simulink model "PMLSM_ThreeLoop_Simple"  (R2026b)
settings: Solver=FixedStepDiscrete  StopTime=12  FixedStep=PMLSM_Ts_s
PreLoadFcn:
  | init_PMLSM_fpga_cosim_params;
InitFcn:
  | reload(get_param('PMLSM_ThreeLoop_Simple','ModelWorkspace'));
values from neighbouring files (symbols this model uses):
  CPU_Clock = 200e6    (= 200000000)    [PMSLM_Init_Params_MBDL4.m]
  FPGA_Cosim_Enable = 1    [init_PMLSM_fpga_cosim_params.m]
  FPGA_Cosim_Input_Mode = 1    [init_PMLSM_fpga_cosim_params.m]
  FPGA_Cosim_Ts_s = 50e-6    (= 5e-05)    [init_PMLSM_fpga_cosim_params.m]
  FPGA_Reference_Mode = 1    [init_PMLSM_step7c_params.m]
  FPGA_Smoke_ia_A = 1.0    (= 1)    [init_PMLSM_fpga_cosim_params.m]
  FPGA_Smoke_ib_A = -0.5    [init_PMLSM_fpga_cosim_params.m]
  FPGA_Smoke_ic_A = -0.5    [init_PMLSM_fpga_cosim_params.m]
  FPGA_Smoke_id_ref_A = 0.0    (= 0)    [init_PMLSM_fpga_cosim_params.m]
  FPGA_Smoke_iq_ref_A = 0.0    (= 0)    [init_PMLSM_fpga_cosim_params.m]
  FPGA_Smoke_theta_rad = 0.0    (= 0)    [init_PMLSM_fpga_cosim_params.m]
  FPGA_Smoke_vdc_V = 48.0    (= 48)    [init_PMLSM_fpga_cosim_params.m]
  FPGA_Smoke_we_radps = 0.0    (= 0)    [init_PMLSM_fpga_cosim_params.m]
  FPGA_TBPRD = 2500    [init_PMLSM_fpga_cosim_params.m]
  Iq_fric_run = 0.05    [PMSLM_Init_Params_MBDL4.m]
  Iq_fric_start = 0.40    (= 0.4)    [PMSLM_Init_Params_MBDL4.m]
  Iq_int_limit = 0.10    (= 0.1)    [PMSLM_Init_Params_MBDL4.m]
  Kaw_d = Kaw_q    (= 0.2)    [PMSLM_Init_Params_MBDL4.m]
  Kaw_q = 0.2    [PMSLM_Init_Params_MBDL4.m]
  Kaw_s = 0.4    [PMSLM_Init_Params_MBDL4.m]
  Ki_ACR = ACR_Commissioning_Scale*Ki_ACR_Baseline    (= 2962.5)    [PMSLM_Init_Params_MBDL4.m]
  Ki_ASR = 0.05    [PMSLM_Init_Params_MBDL4.m]
  Kp_ACR = ACR_Commissioning_Scale*Kp_ACR_Baseline    (= 2.18125)    [PMSLM_Init_Params_MBDL4.m]
  Kp_ASR = 0.03    [PMSLM_Init_Params_MBDL4.m]
  Kp_pos = 5    [PMSLM_Init_Params_MBDL4.m]
  PMLSM_Ld_H = Ld    (= 0.001745)    [PMSLM_Init_Params_MBDL4.m]
  PMLSM_Lq_H = Lq    (= 0.001745)    [PMSLM_Init_Params_MBDL4.m]
  PMLSM_psi_f_Wb = flux    (= 0.141)    [PMSLM_Init_Params_MBDL4.m]
  PMLSM_Rs_ohm = Rs    (= 2.37)    [PMSLM_Init_Params_MBDL4.m]
  Pos_deadband = 0.02    [PMSLM_Init_Params_MBDL4.m]
  Speed_loop_Iq_Limit = Iq_Limit    (= 0.3)    [PMSLM_Init_Params_MBDL4.m]
  Ts = 1 / PWM_Freq    (= 0.0001)    [PMSLM_Init_Params_MBDL4.m]
  Ts_ACR = 1e-4    (= 0.0001)    [PMSLM_Init_Params_MBDL4.m]
  Ts_ASR = 1e-3    (= 0.001)    [PMSLM_Init_Params_MBDL4.m]
  Udc = 48    [PMSLM_Init_Params_MBDL4.m]
  v_ff_eps = 0.5    [PMSLM_Init_Params_MBDL4.m]
  v_over_eps = 3    [PMSLM_Init_Params_MBDL4.m]
  V_pos_max_mmps = 10    [PMSLM_Init_Params_MBDL4.m]
  v_ref_max = 20    [PMSLM_Init_Params_MBDL4.m]
  v_ref_set_step_dn = v_ref_set_rate_dn * Ts    (= 0.005)    [PMSLM_Init_Params_MBDL4.m]
  v_ref_set_step_up = v_ref_set_rate_up * Ts    (= 0.005)    [PMSLM_Init_Params_MBDL4.m]
  v_ref_zero_eps = 0.2    [PMSLM_Init_Params_MBDL4.m]
  v_stick_off = 3.0    (= 3)    [PMSLM_Init_Params_MBDL4.m]
  v_stick_on = 1.0    (= 1)    [PMSLM_Init_Params_MBDL4.m]
undefined symbols (not defined in the file or in its folder): DiscIntNeverNeededParam, Host_Enable_Schedule, Host_Id_A, Host_Iq_A, Host_Iq_Test_Mode, Host_Load_N, Host_PI_Reset_EN, Host_Speed_mmps, Host_Speed_Ramp_s, Host_Start_s, Host_Target_mm, Host_Traj_Amax, Host_Traj_Jmax, Host_Traj_Vmax, PMLSM_Bv_N_per_mps, PMLSM_deadtime_current_eps_A, PMLSM_deadtime_ratio, PMLSM_Fc_N, PMLSM_Kf_peak_N_per_Apeak, PMLSM_M_kg, PMLSM_pwm_period_counts, PMLSM_tau_NN_m, PMLSM_theta_offset_rad, PMLSM_Ts_s, PMLSM_v_eps_mps
libraries: simulink x7, mcbeeMathTransformLib x2, vivadosimlib x1
(part 1 of 2)

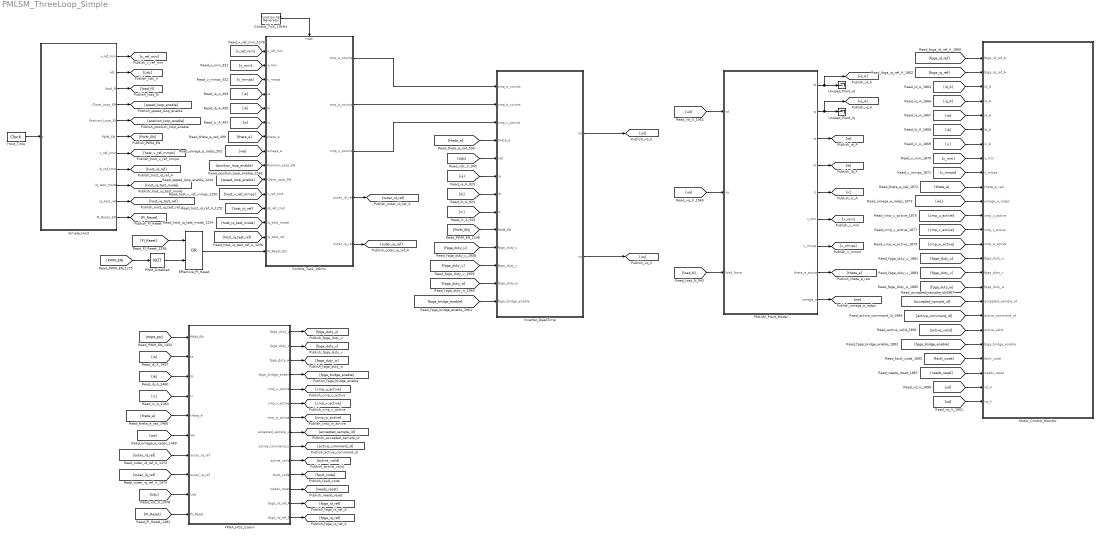
== system PMLSM_ThreeLoop_Simple ==
  Control_Task_10kHz : Subsystem
  Control_Tick_10kHz : FunctionCallGenerator  SampleTime=Ts
  Effective_PI_Reset : Logic  Operator=OR  AllPortsSameDT=off  OutDataTypeStr=boolean
  FPGA_HDL_Cosim : Subsystem
  Host_Time : DigitalClock  SampleTime=Ts_ACR
  Inverter_DeadTime : Subsystem
  Motor_Control_Monitor : Subsystem
  PMLSM_Plant_Model : Subsystem
  PWM_Disabled : Logic  Operator=NOT  AllPortsSameDT=off  OutDataTypeStr=boolean
  Simple_Host : MATLAB Function  TreatAsAtomicUnit=on
  Unused_Plant_Id : Terminator
  Unused_Plant_Iq : Terminator
  wires:
  Host_Time/1 -> Simple_Host/1(t)
  Simple_Host/2(vdc) -> [Udc]
  Simple_Host/3(load_N) -> [load_N]
  Simple_Host/11(PI_Reset_EN) -> [PI_Reset]
  Simple_Host/10(iq_test_ref) -> [host_iq_test_ref]
  Simple_Host/9(iq_test_mode) -> [host_iq_test_mode]
  Simple_Host/8(id_ref_cmd) -> [host_id_ref]
  Simple_Host/7(v_ref_cmd) -> [host_v_ref_mmps]
  Simple_Host/6(PWM_EN) -> [PWM_EN]
  Simple_Host/5(Position_Loop_EN) -> [position_loop_enable]
  Simple_Host/4(Close_Loop_EN) -> [speed_loop_enable]
  [PWM_EN] -> PWM_Disabled/1
  PWM_Disabled/1 -> Effective_PI_Reset/2
  Effective_PI_Reset/1 -> Control_Task_10kHz/15(PI_Reset_EN)
  [speed_loop_enable] -> Control_Task_10kHz/10(Close_Loop_EN)
  [position_loop_enable] -> Control_Task_10kHz/9(Position_Loop_EN)
  [host_v_ref_mmps] -> Control_Task_10kHz/11(v_ref_cmd)
  [host_id_ref] -> Control_Task_10kHz/12(id_ref_cmd)
  [host_iq_test_mode] -> Control_Task_10kHz/13(iq_test_mode)
  [host_iq_test_ref] -> Control_Task_10kHz/14(iq_test_ref)
  [PI_Reset] -> Effective_PI_Reset/1
  Simple_Host/1(x_ref_mm) -> [x_ref_mm]
  [x_mm] -> Control_Task_10kHz/2(x_mm)
  [v_mmps] -> Control_Task_10kHz/3(v_mmps)
  [ia] -> Control_Task_10kHz/4(ia)
  [ib] -> Control_Task_10kHz/5(ib)
  [ic] -> Control_Task_10kHz/6(ic)
  [we] -> Control_Task_10kHz/8(omega_e)
  [theta_e] -> Control_Task_10kHz/7(theta_e)
  Control_Tick_10kHz/1 -> Control_Task_10kHz/Trigger
  [x_ref_mm] -> Control_Task_10kHz/1(x_ref_mm)
  [uq] -> Motor_Control_Monitor/25(vq_V)
  [ud] -> Motor_Control_Monitor/24(vd_V)
  [needs_reset] -> Motor_Control_Monitor/23(needs_reset)
  [fault_code] -> Motor_Control_Monitor/22(fault_code)
  [fpga_bridge_enable] -> Motor_Control_Monitor/21(fpga_bridge_enable)
  [active_valid] -> Motor_Control_Monitor/20(active_valid)
  [active_command_id] -> Motor_Control_Monitor/19(active_command_id)
  [accepted_sample_id] -> Motor_Control_Monitor/18(accepted_sample_id)
  [fpga_duty_w] -> Motor_Control_Monitor/17(fpga_duty_w)
  [fpga_duty_v] -> Motor_Control_Monitor/16(fpga_duty_v)
  [fpga_duty_u] -> Motor_Control_Monitor/15(fpga_duty_u)
  [cmp_w_active] -> Motor_Control_Monitor/14(cmp_w_active)
  [cmp_v_active] -> Motor_Control_Monitor/13(cmp_v_active)
  [cmp_u_active] -> Motor_Control_Monitor/12(cmp_u_active)
  [we] -> Motor_Control_Monitor/11(omega_e_radps)
  [theta_e] -> Motor_Control_Monitor/10(theta_e_rad)
  [v_mmps] -> Motor_Control_Monitor/9(v_mmps)
  [x_mm] -> Motor_Control_Monitor/8(x_mm)
  [ic] -> Motor_Control_Monitor/7(ic_A)
  [ib] -> Motor_Control_Monitor/6(ib_A)
  [ia] -> Motor_Control_Monitor/5(ia_A)
  [iq_A] -> Motor_Control_Monitor/4(iq_A)
  [id_A] -> Motor_Control_Monitor/3(id_A)
  [fpga_iq_ref] -> Motor_Control_Monitor/2(fpga_iq_ref_A)
  [fpga_id_ref] -> Motor_Control_Monitor/1(fpga_id_ref_A)
  FPGA_HDL_Cosim/12(needs_reset) -> [needs_reset]
  FPGA_HDL_Cosim/11(fault_code) -> [fault_code]
  FPGA_HDL_Cosim/10(active_valid) -> [active_valid]
  FPGA_HDL_Cosim/9(active_command_id) -> [active_command_id]
  FPGA_HDL_Cosim/8(accepted_sample_id) -> [accepted_sample_id]
  FPGA_HDL_Cosim/7(cmp_w_active) -> [cmp_w_active]
  FPGA_HDL_Cosim/6(cmp_v_active) -> [cmp_v_active]
  FPGA_HDL_Cosim/5(cmp_u_active) -> [cmp_u_active]
  FPGA_HDL_Cosim/14(fpga_iq_ref_A) -> [fpga_iq_ref]
  FPGA_HDL_Cosim/13(fpga_id_ref_A) -> [fpga_id_ref]
  FPGA_HDL_Cosim/4(fpga_bridge_enable) -> [fpga_bridge_enable]
  FPGA_HDL_Cosim/3(fpga_duty_w) -> [fpga_duty_w]
  FPGA_HDL_Cosim/2(fpga_duty_v) -> [fpga_duty_v]
  FPGA_HDL_Cosim/1(fpga_duty_u) -> [fpga_duty_u]
  [PI_Reset] -> FPGA_HDL_Cosim/10(PI_Reset)
  [Udc] -> FPGA_HDL_Cosim/9(Udc)
  [outer_iq_ref] -> FPGA_HDL_Cosim/8(outer_iq_ref)
  [outer_id_ref] -> FPGA_HDL_Cosim/7(outer_id_ref)
  [we] -> FPGA_HDL_Cosim/6(we)
  [theta_e] -> FPGA_HDL_Cosim/5(theta_e)
  [ic] -> FPGA_HDL_Cosim/4(ic)
  [ib] -> FPGA_HDL_Cosim/3(ib)
  [ia] -> FPGA_HDL_Cosim/2(ia)
  [PWM_EN] -> FPGA_HDL_Cosim/1(PWM_EN)
  PMLSM_Plant_Model/6(x_mm) -> [x_mm]
  PMLSM_Plant_Model/7(v_mmps) -> [v_mmps]
  PMLSM_Plant_Model/3(ia) -> [ia]
  PMLSM_Plant_Model/4(ib) -> [ib]
  PMLSM_Plant_Model/5(ic) -> [ic]
  PMLSM_Plant_Model/8(theta_e_actual) -> [theta_e]
  PMLSM_Plant_Model/9(omega_e) -> [we]
  PMLSM_Plant_Model/1(id) -> Unused_Plant_Id/1, [id_A]
  PMLSM_Plant_Model/2(iq) -> Unused_Plant_Iq/1, [iq_A]
  [load_N] -> PMLSM_Plant_Model/3(load_force)
  Control_Task_10kHz/5(outer_iq_ref) -> [outer_iq_ref]
  Control_Task_10kHz/4(outer_id_ref) -> [outer_id_ref]
  [uq] -> PMLSM_Plant_Model/2(vq)
  [ud] -> PMLSM_Plant_Model/1(vd)
  [fpga_bridge_enable] -> Inverter_DeadTime/13(fpga_bridge_enable)
  [fpga_duty_w] -> Inverter_DeadTime/12(fpga_duty_w)
  [fpga_duty_v] -> Inverter_DeadTime/11(fpga_duty_v)
  [fpga_duty_u] -> Inverter_DeadTime/10(fpga_duty_u)
  [ic] -> Inverter_DeadTime/8(ic)
  [ib] -> Inverter_DeadTime/7(ib)
  [ia] -> Inverter_DeadTime/6(ia)
  [theta_e] -> Inverter_DeadTime/4(theta_e)
  [Udc] -> Inverter_DeadTime/5(vdc)
  Inverter_DeadTime/1(vd) -> [ud]
  Inverter_DeadTime/2(vq) -> [uq]
  [PWM_EN] -> Inverter_DeadTime/9(PWM_EN)
  Control_Task_10kHz/1(cmp_a_counts) -> Inverter_DeadTime/1(cmp_a_counts)
  Control_Task_10kHz/2(cmp_b_counts) -> Inverter_DeadTime/2(cmp_b_counts)
  Control_Task_10kHz/3(cmp_c_counts) -> Inverter_DeadTime/3(cmp_c_counts)

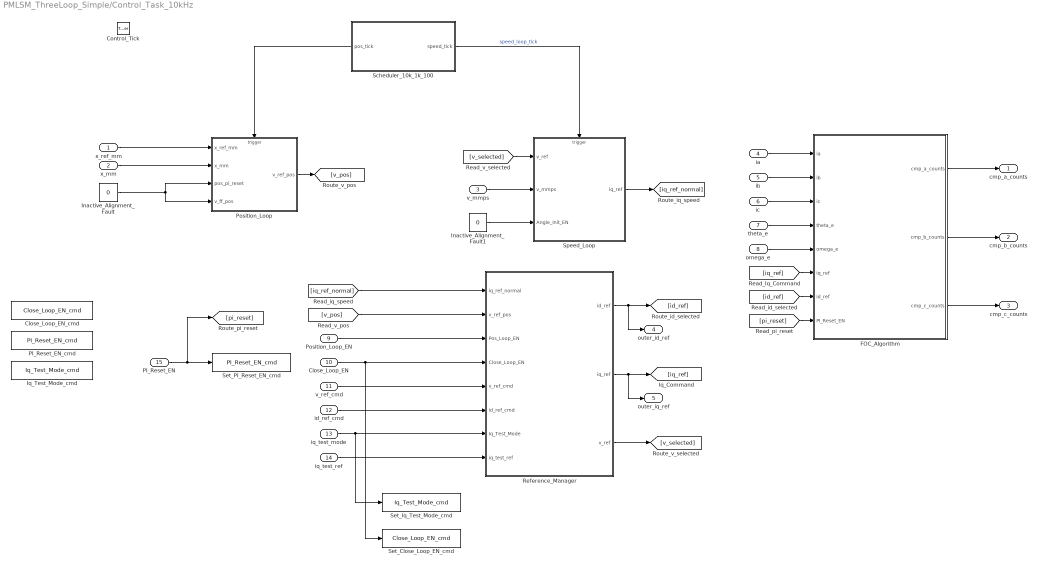
== system PMLSM_ThreeLoop_Simple/Control_Task_10kHz ==
  x_ref_mm : Inport
  x_mm : Inport  Port=2
  v_mmps : Inport  Port=3
  ia : Inport  Port=4
  ib : Inport  Port=5
  ic : Inport  Port=6
  theta_e : Inport  Port=7
  omega_e : Inport  Port=8
  Position_Loop_EN : Inport  Port=9
  Close_Loop_EN : Inport  Port=10
  v_ref_cmd : Inport  Port=11
  id_ref_cmd : Inport  Port=12
  iq_test_mode : Inport  Port=13
  iq_test_ref : Inport  Port=14
  PI_Reset_EN : Inport  Port=15
  Control_Tick : TriggerPort  TriggerType=function-call  VariantControl=(inherit)  PortDimensions=1
  Close_Loop_EN_cmd : DataStoreMemory  DataStoreName=Close_Loop_EN_cmd  WriteAfterWriteMsg=warning  InitialValue=1  ShowAdditionalParam=off
  FOC_Algorithm : Subsystem
  Inactive_Alignment_Fault : Constant  Value=0
  Inactive_Alignment_Fault1 : Constant  Value=0
  Iq_Test_Mode_cmd : DataStoreMemory  DataStoreName=Iq_Test_Mode_cmd  WriteAfterWriteMsg=warning  ShowAdditionalParam=off
  PI_Reset_EN_cmd : DataStoreMemory  DataStoreName=PI_Reset_EN_cmd  WriteAfterWriteMsg=warning  ShowAdditionalParam=off
  Position_Loop : Subsystem  TreatAsAtomicUnit=on
  Reference_Manager : Subsystem
  Scheduler_10k_1k_100 : Subsystem
  Set_Close_Loop_EN_cmd : DataStoreWrite  Priority=-10  DataStoreName=Close_Loop_EN_cmd  IndexOptions=Index vector (dialog)  Indices=1  OutputSizes=1
  Set_Iq_Test_Mode_cmd : DataStoreWrite  Priority=-10  DataStoreName=Iq_Test_Mode_cmd  IndexOptions=Index vector (dialog)  Indices=1  OutputSizes=1
  Set_PI_Reset_EN_cmd : DataStoreWrite  Priority=-10  DataStoreName=PI_Reset_EN_cmd  IndexOptions=Index vector (dialog)  Indices=1  OutputSizes=1
  Speed_Loop : Subsystem  TreatAsAtomicUnit=on
  cmp_a_counts : Outport
  cmp_b_counts : Outport  Port=2
  cmp_c_counts : Outport  Port=3
  outer_id_ref : Outport  Port=4
  outer_iq_ref : Outport  Port=5
  wires:
  [iq_ref] -> FOC_Algorithm/6(iq_ref)
  FOC_Algorithm/3(cmp_c_counts) -> cmp_c_counts/1
  FOC_Algorithm/2(cmp_b_counts) -> cmp_b_counts/1
  FOC_Algorithm/1(cmp_a_counts) -> cmp_a_counts/1
  omega_e/1 -> FOC_Algorithm/5(omega_e)
  theta_e/1 -> FOC_Algorithm/4(theta_e)
  ic/1 -> FOC_Algorithm/3(ic)
  ib/1 -> FOC_Algorithm/2(ib)
  ia/1 -> FOC_Algorithm/1(ia)
  iq_test_ref/1 -> Reference_Manager/8(iq_test_ref)
  id_ref_cmd/1 -> Reference_Manager/6(id_ref_cmd)
  v_ref_cmd/1 -> Reference_Manager/5(v_ref_cmd)
  Position_Loop_EN/1 -> Reference_Manager/3(Pos_Loop_EN)
  [pi_reset] -> FOC_Algorithm/8(PI_Reset_EN)
  [id_ref] -> FOC_Algorithm/7(id_ref)
  [v_selected] -> Speed_Loop/1(v_ref)
  [iq_ref_normal] -> Reference_Manager/1(iq_ref_normal)
  [v_pos] -> Reference_Manager/2(v_ref_pos)
  Reference_Manager/3(v_ref) -> [v_selected]
  Inactive_Alignment_Fault/1 -> Position_Loop/3(pos_pi_reset), Position_Loop/4(v_ff_pos)
  Speed_Loop/1(iq_ref) -> [iq_ref_normal]
  Position_Loop/1(v_ref_pos) -> [v_pos]
  x_mm/1 -> Position_Loop/2(x_mm)
  x_ref_mm/1 -> Position_Loop/1(x_ref_mm)
  Scheduler_10k_1k_100/1(speed_tick) -> Speed_Loop/Trigger  "speed_loop_tick"
  Scheduler_10k_1k_100/2(pos_tick) -> Position_Loop/Trigger
  PI_Reset_EN/1 -> [pi_reset], Set_PI_Reset_EN_cmd/1
  iq_test_mode/1 -> Set_Iq_Test_Mode_cmd/1, Reference_Manager/7(Iq_Test_Mode)
  Close_Loop_EN/1 -> Set_Close_Loop_EN_cmd/1, Reference_Manager/4(Close_Loop_EN)
  Inactive_Alignment_Fault1/1 -> Speed_Loop/3(Angle_Init_EN)
  v_mmps/1 -> Speed_Loop/2(v_mmps)
  Reference_Manager/1(id_ref) -> outer_id_ref/1, [id_ref]
  Reference_Manager/2(iq_ref) -> outer_iq_ref/1, [iq_ref]

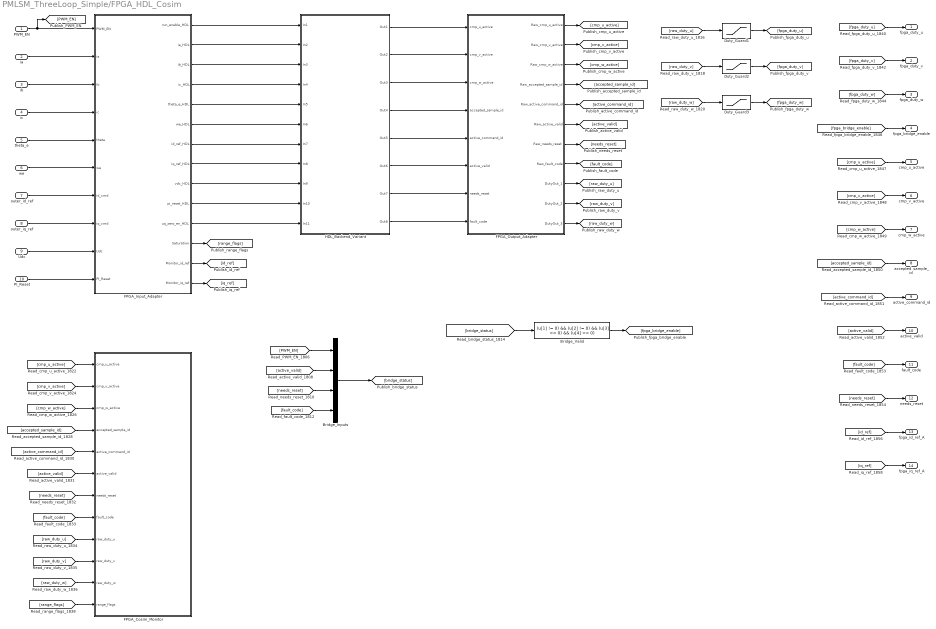
== system PMLSM_ThreeLoop_Simple/FPGA_HDL_Cosim ==
  PWM_EN : Inport
  ia : Inport  Port=2
  ib : Inport  Port=3
  ic : Inport  Port=4
  theta_e : Inport  Port=5
  we : Inport  Port=6
  outer_id_ref : Inport  Port=7
  outer_iq_ref : Inport  Port=8
  Udc : Inport  Port=9
  PI_Reset : Inport  Port=10
  Bridge_Inputs : Mux
  Bridge_Valid : Fcn  Expr=(u[1] != 0) && (u[2] != 0) && (u[3] == 0) && (u[4] == 0)
  Duty_Guard1 : Saturate  UpperLimit=1  LowerLimit=0
  Duty_Guard2 : Saturate  UpperLimit=1  LowerLimit=0
  Duty_Guard3 : Saturate  UpperLimit=1  LowerLimit=0
  FPGA_Cosim_Monitor : Subsystem
  FPGA_Input_Adapter : Subsystem
  FPGA_Output_Adapter : Subsystem
  HDL_Backend_Variant : Subsystem  Variant=on
  fpga_duty_u : Outport
  fpga_duty_v : Outport  Port=2
  fpga_duty_w : Outport  Port=3
  fpga_bridge_enable : Outport  Port=4
  cmp_u_active : Outport  Port=5
  cmp_v_active : Outport  Port=6
  cmp_w_active : Outport  Port=7
  accepted_sample_id : Outport  Port=8
  active_command_id : Outport  Port=9
  active_valid : Outport  Port=10
  fault_code : Outport  Port=11
  needs_reset : Outport  Port=12
  fpga_id_ref_A : Outport  Port=13
  fpga_iq_ref_A : Outport  Port=14
  wires:
  ia/1 -> FPGA_Input_Adapter/2(ia)
  ib/1 -> FPGA_Input_Adapter/3(ib)
  ic/1 -> FPGA_Input_Adapter/4(ic)
  theta_e/1 -> FPGA_Input_Adapter/5(theta)
  we/1 -> FPGA_Input_Adapter/6(we)
  outer_id_ref/1 -> FPGA_Input_Adapter/7(id_cmd)
  outer_iq_ref/1 -> FPGA_Input_Adapter/8(iq_cmd)
  Udc/1 -> FPGA_Input_Adapter/9(Udc)
  PI_Reset/1 -> FPGA_Input_Adapter/10(PI_Reset)
  FPGA_Input_Adapter/1(run_enable_HDL) -> HDL_Backend_Variant/1(In1)
  FPGA_Input_Adapter/2(ia_HDL) -> HDL_Backend_Variant/2(In2)
  FPGA_Input_Adapter/3(ib_HDL) -> HDL_Backend_Variant/3(In3)
  FPGA_Input_Adapter/4(ic_HDL) -> HDL_Backend_Variant/4(In4)
  FPGA_Input_Adapter/5(theta_e_HDL) -> HDL_Backend_Variant/5(In5)
  FPGA_Input_Adapter/6(we_HDL) -> HDL_Backend_Variant/6(In6)
  FPGA_Input_Adapter/7(id_ref_HDL) -> HDL_Backend_Variant/7(In7)
  FPGA_Input_Adapter/8(iq_ref_HDL) -> HDL_Backend_Variant/8(In8)
  FPGA_Input_Adapter/9(vdc_HDL) -> HDL_Backend_Variant/9(In9)
  FPGA_Input_Adapter/10(pi_reset_HDL) -> HDL_Backend_Variant/10(In10)
  FPGA_Input_Adapter/11(uq_zero_en_HDL) -> HDL_Backend_Variant/11(In11)
  [iq_ref] -> fpga_iq_ref_A/1
  [id_ref] -> fpga_id_ref_A/1
  [needs_reset] -> needs_reset/1
  [fault_code] -> fault_code/1
  [active_valid] -> active_valid/1
  [active_command_id] -> active_command_id/1
  [accepted_sample_id] -> accepted_sample_id/1
  [cmp_w_active] -> cmp_w_active/1
  [cmp_v_active] -> cmp_v_active/1
  [cmp_u_active] -> cmp_u_active/1
  [fpga_bridge_enable] -> fpga_bridge_enable/1
  [fpga_duty_w] -> fpga_duty_w/1
  [fpga_duty_v] -> fpga_duty_v/1
  [fpga_duty_u] -> fpga_duty_u/1
  [range_flags] -> FPGA_Cosim_Monitor/12(range_flags)
  [raw_duty_w] -> FPGA_Cosim_Monitor/11(raw_duty_w)
  [raw_duty_v] -> FPGA_Cosim_Monitor/10(raw_duty_v)
  [raw_duty_u] -> FPGA_Cosim_Monitor/9(raw_duty_u)
  [fault_code] -> FPGA_Cosim_Monitor/8(fault_code)
  [needs_reset] -> FPGA_Cosim_Monitor/7(needs_reset)
  [active_valid] -> FPGA_Cosim_Monitor/6(active_valid)
  [active_command_id] -> FPGA_Cosim_Monitor/5(active_command_id)
  [accepted_sample_id] -> FPGA_Cosim_Monitor/4(accepted_sample_id)
  [cmp_w_active] -> FPGA_Cosim_Monitor/3(cmp_w_active)
  [cmp_v_active] -> FPGA_Cosim_Monitor/2(cmp_v_active)
  [cmp_u_active] -> FPGA_Cosim_Monitor/1(cmp_u_active)
  [raw_duty_w] -> Duty_Guard3/1
  [raw_duty_v] -> Duty_Guard2/1
  [raw_duty_u] -> Duty_Guard1/1
  [bridge_status] -> Bridge_Valid/1
  [fault_code] -> Bridge_Inputs/4
  [needs_reset] -> Bridge_Inputs/3
  [active_valid] -> Bridge_Inputs/2
  [PWM_EN] -> Bridge_Inputs/1
  FPGA_Input_Adapter/14(Monitor_iq_ref) -> [iq_ref]
  FPGA_Input_Adapter/13(Monitor_id_ref) -> [id_ref]
  Bridge_Valid/1 -> [fpga_bridge_enable]
  Bridge_Inputs/1 -> [bridge_status]
  Duty_Guard3/1 -> [fpga_duty_w]
  Duty_Guard2/1 -> [fpga_duty_v]
  Duty_Guard1/1 -> [fpga_duty_u]
  HDL_Backend_Variant/8(Out8) -> FPGA_Output_Adapter/8(fault_code)
  HDL_Backend_Variant/7(Out7) -> FPGA_Output_Adapter/7(needs_reset)
  HDL_Backend_Variant/6(Out6) -> FPGA_Output_Adapter/6(active_valid)
  HDL_Backend_Variant/5(Out5) -> FPGA_Output_Adapter/5(active_command_id)
  HDL_Backend_Variant/4(Out4) -> FPGA_Output_Adapter/4(accepted_sample_id)
  HDL_Backend_Variant/3(Out3) -> FPGA_Output_Adapter/3(cmp_w_active)
  HDL_Backend_Variant/2(Out2) -> FPGA_Output_Adapter/2(cmp_v_active)
  HDL_Backend_Variant/1(Out1) -> FPGA_Output_Adapter/1(cmp_u_active)
  FPGA_Input_Adapter/12(Saturation) -> [range_flags]
  FPGA_Output_Adapter/11(DutyOut_3) -> [raw_duty_w]
  FPGA_Output_Adapter/10(DutyOut_2) -> [raw_duty_v]
  FPGA_Output_Adapter/9(DutyOut_1) -> [raw_duty_u]
  FPGA_Output_Adapter/8(Raw_fault_code) -> [fault_code]
  FPGA_Output_Adapter/7(Raw_needs_reset) -> [needs_reset]
  FPGA_Output_Adapter/6(Raw_active_valid) -> [active_valid]
  FPGA_Output_Adapter/5(Raw_active_command_id) -> [active_command_id]
  FPGA_Output_Adapter/4(Raw_accepted_sample_id) -> [accepted_sample_id]
  FPGA_Output_Adapter/3(Raw_cmp_w_active) -> [cmp_w_active]
  FPGA_Output_Adapter/2(Raw_cmp_v_active) -> [cmp_v_active]
  FPGA_Output_Adapter/1(Raw_cmp_u_active) -> [cmp_u_active]
  PWM_EN/1 -> [PWM_EN], FPGA_Input_Adapter/1(PWM_EN)

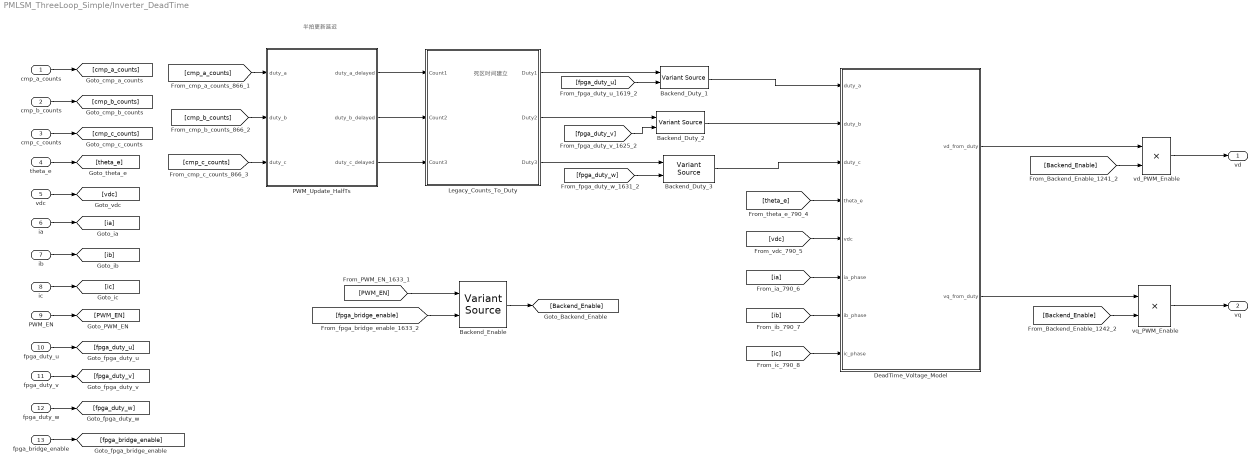
== system PMLSM_ThreeLoop_Simple/Inverter_DeadTime ==
  note: 死区时间建立
  note: 半拍更新延迟
  cmp_a_counts : Inport
  cmp_b_counts : Inport  Port=2
  cmp_c_counts : Inport  Port=3
  theta_e : Inport  Port=4
  vdc : Inport  Port=5
  ia : Inport  Port=6
  ib : Inport  Port=7
  ic : Inport  Port=8
  PWM_EN : Inport  Port=9
  fpga_duty_u : Inport  Port=10
  fpga_duty_v : Inport  Port=11
  fpga_duty_w : Inport  Port=12
  fpga_bridge_enable : Inport  Port=13
  Backend_Duty_1 : VariantSource  VariantControls={V_Backend_Legacy, V_Backend_FPGA}
  Backend_Duty_2 : VariantSource  VariantControls={V_Backend_Legacy, V_Backend_FPGA}
  Backend_Duty_3 : VariantSource  VariantControls={V_Backend_Legacy, V_Backend_FPGA}
  Backend_Enable : VariantSource  VariantControls={V_Backend_Legacy, V_Backend_FPGA}
  DeadTime_Voltage_Model : Subsystem
  Legacy_Counts_To_Duty : Subsystem
  PWM_Update_HalfTs : Subsystem
  vd_PWM_Enable : Product  Inputs=**
  vq_PWM_Enable : Product  Inputs=**
  vd : Outport
  vq : Outport  Port=2
  wires:
  [fpga_bridge_enable] -> Backend_Enable/2
  [fpga_duty_w] -> Backend_Duty_3/2
  [fpga_duty_v] -> Backend_Duty_2/2
  [fpga_duty_u] -> Backend_Duty_1/2
  [PWM_EN] -> Backend_Enable/1
  [ic] -> DeadTime_Voltage_Model/8(ic_phase)
  [ib] -> DeadTime_Voltage_Model/7(ib_phase)
  [ia] -> DeadTime_Voltage_Model/6(ia_phase)
  [vdc] -> DeadTime_Voltage_Model/5(vdc)
  [theta_e] -> DeadTime_Voltage_Model/4(theta_e)
  [cmp_c_counts] -> PWM_Update_HalfTs/3(duty_c)
  [cmp_b_counts] -> PWM_Update_HalfTs/2(duty_b)
  [cmp_a_counts] -> PWM_Update_HalfTs/1(duty_a)
  fpga_bridge_enable/1 -> [fpga_bridge_enable]
  PWM_EN/1 -> [PWM_EN]
  Backend_Duty_3/1 -> DeadTime_Voltage_Model/3(duty_c)
  fpga_duty_w/1 -> [fpga_duty_w]
  Legacy_Counts_To_Duty/3(Duty3) -> Backend_Duty_3/1
  PWM_Update_HalfTs/3(duty_c_delayed) -> Legacy_Counts_To_Duty/3(Count3)
  Backend_Duty_2/1 -> DeadTime_Voltage_Model/2(duty_b)
  fpga_duty_v/1 -> [fpga_duty_v]
  Legacy_Counts_To_Duty/2(Duty2) -> Backend_Duty_2/1
  PWM_Update_HalfTs/2(duty_b_delayed) -> Legacy_Counts_To_Duty/2(Count2)
  Backend_Duty_1/1 -> DeadTime_Voltage_Model/1(duty_a)
  fpga_duty_u/1 -> [fpga_duty_u]
  Legacy_Counts_To_Duty/1(Duty1) -> Backend_Duty_1/1
  PWM_Update_HalfTs/1(duty_a_delayed) -> Legacy_Counts_To_Duty/1(Count1)
  ic/1 -> [ic]
  ib/1 -> [ib]
  ia/1 -> [ia]
  vdc/1 -> [vdc]
  theta_e/1 -> [theta_e]
  cmp_a_counts/1 -> [cmp_a_counts]
  cmp_b_counts/1 -> [cmp_b_counts]
  cmp_c_counts/1 -> [cmp_c_counts]
  [Backend_Enable] -> vd_PWM_Enable/2
  [Backend_Enable] -> vq_PWM_Enable/2
  DeadTime_Voltage_Model/1(vd_from_duty) -> vd_PWM_Enable/1
  DeadTime_Voltage_Model/2(vq_from_duty) -> vq_PWM_Enable/1
  Backend_Enable/1 -> [Backend_Enable]
  vd_PWM_Enable/1 -> vd/1
  vq_PWM_Enable/1 -> vq/1

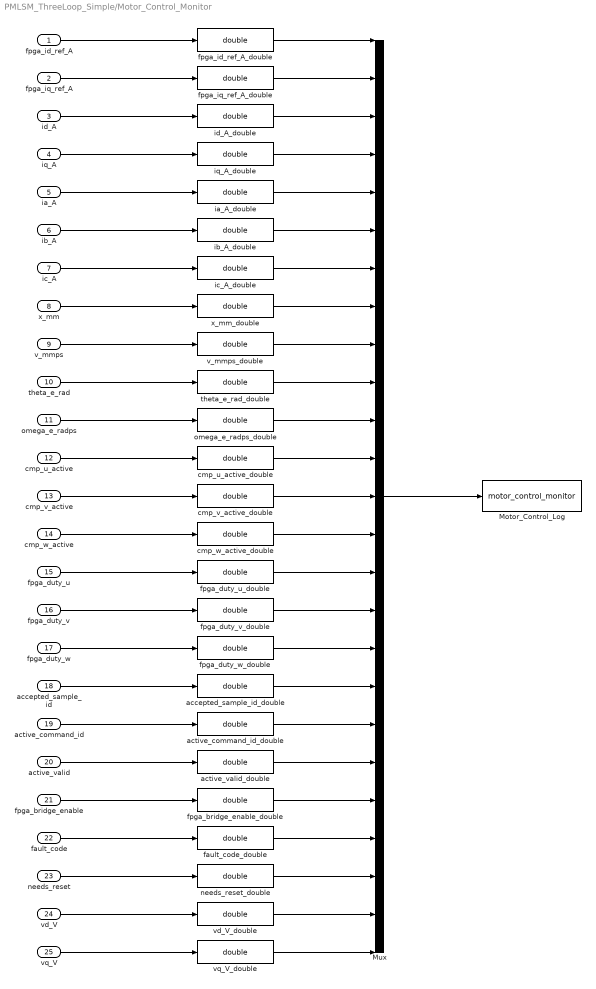
== system PMLSM_ThreeLoop_Simple/Motor_Control_Monitor ==
  fpga_id_ref_A : Inport
  fpga_iq_ref_A : Inport  Port=2
  id_A : Inport  Port=3
  iq_A : Inport  Port=4
  ia_A : Inport  Port=5
  ib_A : Inport  Port=6
  ic_A : Inport  Port=7
  x_mm : Inport  Port=8
  v_mmps : Inport  Port=9
  theta_e_rad : Inport  Port=10
  omega_e_radps : Inport  Port=11
  cmp_u_active : Inport  Port=12
  cmp_v_active : Inport  Port=13
  cmp_w_active : Inport  Port=14
  fpga_duty_u : Inport  Port=15
  fpga_duty_v : Inport  Port=16
  fpga_duty_w : Inport  Port=17
  accepted_sample_id : Inport  Port=18
  active_command_id : Inport  Port=19
  active_valid : Inport  Port=20
  fpga_bridge_enable : Inport  Port=21
  fault_code : Inport  Port=22
  needs_reset : Inport  Port=23
  vd_V : Inport  Port=24
  vq_V : Inport  Port=25
  Motor_Control_Log : ToWorkspace  VariableName=motor_control_monitor  SaveFormat=Timeseries  SampleTime=-1
  Mux : Mux  Inputs=25
  accepted_sample_id_double : DataTypeConversion  OutDataTypeStr=double  SaturateOnIntegerOverflow=off  RndMeth=Floor
  active_command_id_double : DataTypeConversion  OutDataTypeStr=double  SaturateOnIntegerOverflow=off  RndMeth=Floor
  active_valid_double : DataTypeConversion  OutDataTypeStr=double  SaturateOnIntegerOverflow=off  RndMeth=Floor
  cmp_u_active_double : DataTypeConversion  OutDataTypeStr=double  SaturateOnIntegerOverflow=off  RndMeth=Floor
  cmp_v_active_double : DataTypeConversion  OutDataTypeStr=double  SaturateOnIntegerOverflow=off  RndMeth=Floor
  cmp_w_active_double : DataTypeConversion  OutDataTypeStr=double  SaturateOnIntegerOverflow=off  RndMeth=Floor
  fault_code_double : DataTypeConversion  OutDataTypeStr=double  SaturateOnIntegerOverflow=off  RndMeth=Floor
  fpga_bridge_enable_double : DataTypeConversion  OutDataTypeStr=double  SaturateOnIntegerOverflow=off  RndMeth=Floor
  fpga_duty_u_double : DataTypeConversion  OutDataTypeStr=double  SaturateOnIntegerOverflow=off  RndMeth=Floor
  fpga_duty_v_double : DataTypeConversion  OutDataTypeStr=double  SaturateOnIntegerOverflow=off  RndMeth=Floor
  fpga_duty_w_double : DataTypeConversion  OutDataTypeStr=double  SaturateOnIntegerOverflow=off  RndMeth=Floor
  fpga_id_ref_A_double : DataTypeConversion  OutDataTypeStr=double  SaturateOnIntegerOverflow=off  RndMeth=Floor
  fpga_iq_ref_A_double : DataTypeConversion  OutDataTypeStr=double  SaturateOnIntegerOverflow=off  RndMeth=Floor
  ia_A_double : DataTypeConversion  OutDataTypeStr=double  SaturateOnIntegerOverflow=off  RndMeth=Floor
  ib_A_double : DataTypeConversion  OutDataTypeStr=double  SaturateOnIntegerOverflow=off  RndMeth=Floor
  ic_A_double : DataTypeConversion  OutDataTypeStr=double  SaturateOnIntegerOverflow=off  RndMeth=Floor
  id_A_double : DataTypeConversion  OutDataTypeStr=double  SaturateOnIntegerOverflow=off  RndMeth=Floor
  iq_A_double : DataTypeConversion  OutDataTypeStr=double  SaturateOnIntegerOverflow=off  RndMeth=Floor
  needs_reset_double : DataTypeConversion  OutDataTypeStr=double  SaturateOnIntegerOverflow=off  RndMeth=Floor
  omega_e_radps_double : DataTypeConversion  OutDataTypeStr=double  SaturateOnIntegerOverflow=off  RndMeth=Floor
  theta_e_rad_double : DataTypeConversion  OutDataTypeStr=double  SaturateOnIntegerOverflow=off  RndMeth=Floor
  v_mmps_double : DataTypeConversion  OutDataTypeStr=double  SaturateOnIntegerOverflow=off  RndMeth=Floor
  vd_V_double : DataTypeConversion  OutDataTypeStr=double  SaturateOnIntegerOverflow=off  RndMeth=Floor
  vq_V_double : DataTypeConversion  OutDataTypeStr=double  SaturateOnIntegerOverflow=off  RndMeth=Floor
  x_mm_double : DataTypeConversion  OutDataTypeStr=double  SaturateOnIntegerOverflow=off  RndMeth=Floor
  wires:
  Mux/1 -> Motor_Control_Log/1
  fpga_id_ref_A/1 -> fpga_id_ref_A_double/1
  fpga_id_ref_A_double/1 -> Mux/1
  fpga_iq_ref_A/1 -> fpga_iq_ref_A_double/1
  fpga_iq_ref_A_double/1 -> Mux/2
  id_A/1 -> id_A_double/1
  id_A_double/1 -> Mux/3
  iq_A/1 -> iq_A_double/1
  iq_A_double/1 -> Mux/4
  ia_A/1 -> ia_A_double/1
  ia_A_double/1 -> Mux/5
  ib_A/1 -> ib_A_double/1
  ib_A_double/1 -> Mux/6
  ic_A/1 -> ic_A_double/1
  ic_A_double/1 -> Mux/7
  x_mm/1 -> x_mm_double/1
  x_mm_double/1 -> Mux/8
  v_mmps/1 -> v_mmps_double/1
  v_mmps_double/1 -> Mux/9
  theta_e_rad/1 -> theta_e_rad_double/1
  theta_e_rad_double/1 -> Mux/10
  omega_e_radps/1 -> omega_e_radps_double/1
  omega_e_radps_double/1 -> Mux/11
  cmp_u_active/1 -> cmp_u_active_double/1
  cmp_u_active_double/1 -> Mux/12
  cmp_v_active/1 -> cmp_v_active_double/1
  cmp_v_active_double/1 -> Mux/13
  cmp_w_active/1 -> cmp_w_active_double/1
  cmp_w_active_double/1 -> Mux/14
  fpga_duty_u/1 -> fpga_duty_u_double/1
  fpga_duty_u_double/1 -> Mux/15
  fpga_duty_v/1 -> fpga_duty_v_double/1
  fpga_duty_v_double/1 -> Mux/16
  fpga_duty_w/1 -> fpga_duty_w_double/1
  fpga_duty_w_double/1 -> Mux/17
  accepted_sample_id/1 -> accepted_sample_id_double/1
  accepted_sample_id_double/1 -> Mux/18
  active_command_id/1 -> active_command_id_double/1
  active_command_id_double/1 -> Mux/19
  active_valid/1 -> active_valid_double/1
  active_valid_double/1 -> Mux/20
  fpga_bridge_enable/1 -> fpga_bridge_enable_double/1
  fpga_bridge_enable_double/1 -> Mux/21
  fault_code/1 -> fault_code_double/1
  fault_code_double/1 -> Mux/22
  needs_reset/1 -> needs_reset_double/1
  needs_reset_double/1 -> Mux/23
  vd_V/1 -> vd_V_double/1
  vd_V_double/1 -> Mux/24
  vq_V/1 -> vq_V_double/1
  vq_V_double/1 -> Mux/25

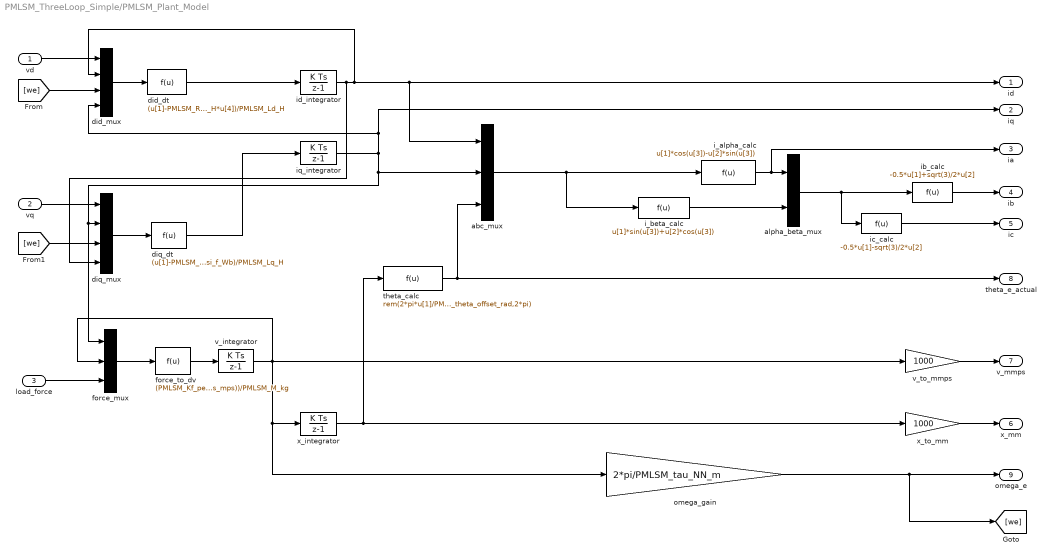
== system PMLSM_ThreeLoop_Simple/PMLSM_Plant_Model ==
  vd : Inport
  vq : Inport  Port=2
  load_force : Inport  Port=3
  abc_mux : Mux  Inputs=3
  alpha_beta_mux : Mux  Inputs=2
  did_dt : Fcn  Expr=(u[1]-PMLSM_Rs_ohm*u[2]+u[3]*PMLSM_Lq_H*u[4])/PMLSM_Ld_H
  did_mux : Mux
  diq_dt : Fcn  Expr=(u[1]-PMLSM_Rs_ohm*u[2]-u[3]*PMLSM_Ld_H*u[4]-u[3]*PMLSM_psi_f_Wb)/PMLSM_Lq_H
  diq_mux : Mux
  force_mux : Mux  Inputs=3
  force_to_dv : Fcn  Expr=(PMLSM_Kf_peak_N_per_Apeak*u[1]-u[3]-PMLSM_Bv_N_per_mps*u[2]-PMLSM_Fc_N*tanh(u[2]/PMLSM_v_eps_mps))/PMLSM_M_kg
  i_alpha_calc : Fcn  Expr=u[1]*cos(u[3])-u[2]*sin(u[3])
  i_beta_calc : Fcn  Expr=u[1]*sin(u[3])+u[2]*cos(u[3])
  ib_calc : Fcn  Expr=-0.5*u[1]+sqrt(3)/2*u[2]
  ic_calc : Fcn  Expr=-0.5*u[1]-sqrt(3)/2*u[2]
  id_integrator : DiscreteIntegrator  gainval=1  SampleTime=PMLSM_Ts_s  ICPrevOutput=DiscIntNeverNeededParam  ICPrevScaledInput=DiscIntNeverNeededParam
  iq_integrator : DiscreteIntegrator  gainval=1  SampleTime=PMLSM_Ts_s  ICPrevOutput=DiscIntNeverNeededParam  ICPrevScaledInput=DiscIntNeverNeededParam
  omega_gain : Gain  Gain=2*pi/PMLSM_tau_NN_m
  theta_calc : Fcn  Expr=rem(2*pi*u[1]/PMLSM_tau_NN_m+PMLSM_theta_offset_rad,2*pi)
  v_integrator : DiscreteIntegrator  gainval=1  SampleTime=PMLSM_Ts_s  ICPrevOutput=DiscIntNeverNeededParam  ICPrevScaledInput=DiscIntNeverNeededParam
  v_to_mmps : Gain  Gain=1000
  x_integrator : DiscreteIntegrator  gainval=1  SampleTime=PMLSM_Ts_s  ICPrevOutput=DiscIntNeverNeededParam  ICPrevScaledInput=DiscIntNeverNeededParam
  x_to_mm : Gain  Gain=1000
  id : Outport
  iq : Outport  Port=2
  ia : Outport  Port=3
  ib : Outport  Port=4
  ic : Outport  Port=5
  x_mm : Outport  Port=6
  v_mmps : Outport  Port=7
  theta_e_actual : Outport  Port=8
  omega_e : Outport  Port=9
  wires:
  ic_calc/1 -> ic/1
  ib_calc/1 -> ib/1
  alpha_beta_mux/1 -> ic_calc/1, ib_calc/1
  i_beta_calc/1 -> alpha_beta_mux/2
  i_alpha_calc/1 -> alpha_beta_mux/1, ia/1
  force_to_dv/1 -> v_integrator/1
  force_mux/1 -> force_to_dv/1
  load_force/1 -> force_mux/3
  diq_dt/1 -> iq_integrator/1
  diq_mux/1 -> diq_dt/1
  vq/1 -> diq_mux/1
  did_dt/1 -> id_integrator/1
  did_mux/1 -> did_dt/1
  vd/1 -> did_mux/1
  x_to_mm/1 -> x_mm/1
  v_to_mmps/1 -> v_mmps/1
  theta_calc/1 -> theta_e_actual/1, abc_mux/3
  omega_gain/1 -> [we], omega_e/1
  id_integrator/1 -> id/1, abc_mux/1, did_mux/2, diq_mux/4
  iq_integrator/1 -> abc_mux/2, force_mux/1, diq_mux/2, iq/1, did_mux/4
  v_integrator/1 -> omega_gain/1, x_integrator/1, v_to_mmps/1, force_mux/2
  x_integrator/1 -> theta_calc/1, x_to_mm/1
  abc_mux/1 -> i_alpha_calc/1, i_beta_calc/1
  [we] -> did_mux/3
  [we] -> diq_mux/3

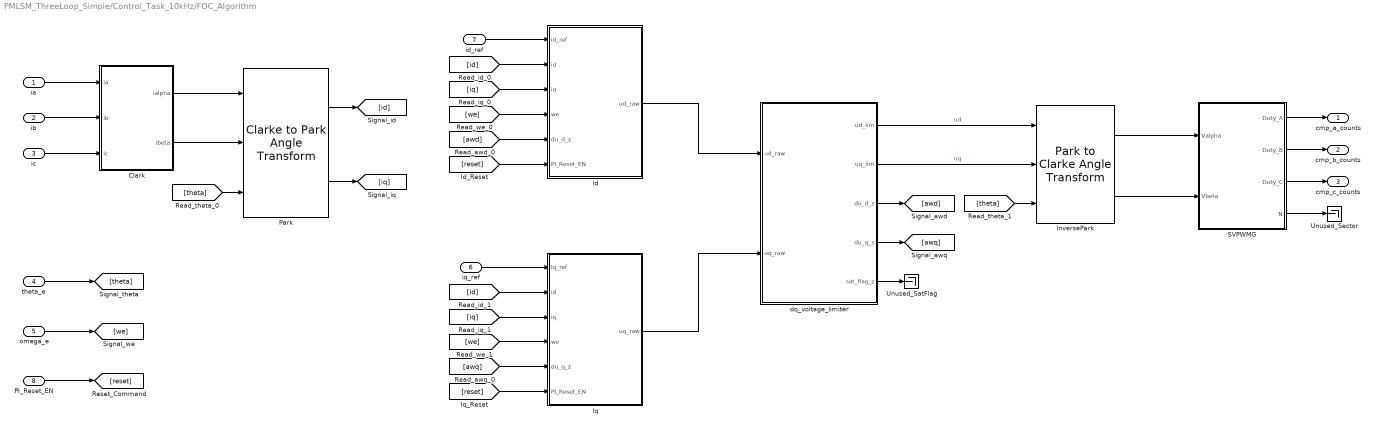
== system PMLSM_ThreeLoop_Simple/Control_Task_10kHz/FOC_Algorithm ==
  ia : Inport
  ib : Inport  Port=2
  ic : Inport  Port=3
  theta_e : Inport  Port=4
  omega_e : Inport  Port=5
  iq_ref : Inport  Port=6
  id_ref : Inport  Port=7
  PI_Reset_EN : Inport  Port=8
  Clark : Subsystem  TreatAsAtomicUnit=on  RTWFcnName=Clack_Fun
  Id : Subsystem  TreatAsAtomicUnit=on  RTWFcnName=Id_Fun
  InversePark : mcbeeMathTransformLib/Park to Clarke Angle Transform  AxisAlignment=D-axis  UseWithEmbedded=on  PhaseInput=Two inputs  ThetaInput=Electrical position  AngleInput=Radians  N_points=1024
  Iq : Subsystem  TreatAsAtomicUnit=on  RTWFcnName=Iq_Fun
  Park : mcbeeMathTransformLib/Clarke to Park Angle Transform  AxisAlignment=D-axis  UseWithEmbedded=on  PhaseInput=Two inputs  ThetaInput=Electrical position  AngleInput=Radians  N_points=1024
  SVPWMG : Subsystem  TreatAsAtomicUnit=on  RTWFcnName=SVPWM_Gen_Fun
  Unused_SatFlag : Terminator
  Unused_Sector : Terminator
  dq_voltage_limiter : Subsystem
  cmp_a_counts : Outport
  cmp_b_counts : Outport  Port=2
  cmp_c_counts : Outport  Port=3
  wires:
  SVPWMG/4("N ") -> Unused_Sector/1
  SVPWMG/3(Duty_C) -> cmp_c_counts/1
  SVPWMG/2(Duty_B) -> cmp_b_counts/1
  SVPWMG/1(Duty_A) -> cmp_a_counts/1
  ic/1 -> Clark/3(ic)
  ib/1 -> Clark/2(ib)
  ia/1 -> Clark/1(ia)
  [theta] -> InversePark/3
  [theta] -> Park/3
  Clark/1(ialpha) -> Park/1
  Clark/2(ibeta) -> Park/2
  theta_e/1 -> [theta]
  Park/1 -> [id]
  Park/2 -> [iq]
  omega_e/1 -> [we]
  dq_voltage_limiter/3(du_d_z) -> [awd]
  dq_voltage_limiter/4(du_q_z) -> [awq]
  dq_voltage_limiter/5(sat_flag_z) -> Unused_SatFlag/1
  dq_voltage_limiter/1(ud_lim) -> InversePark/1  "ud"
  dq_voltage_limiter/2(uq_lim) -> InversePark/2  "uq"
  InversePark/1 -> SVPWMG/1(Valpha)
  InversePark/2 -> SVPWMG/2(Vbeta)
  [reset] -> Iq/6(PI_Reset_EN)
  [reset] -> Id/6(PI_Reset_EN)
  id_ref/1 -> Id/1(id_ref)
  PI_Reset_EN/1 -> [reset]
  Iq/1(uq_raw) -> dq_voltage_limiter/2(uq_raw)
  Id/1(ud_raw) -> dq_voltage_limiter/1(ud_raw)
  iq_ref/1 -> Iq/1(Iq_ref)
  [id] -> Id/2(id)
  [id] -> Iq/2(id)
  [iq] -> Id/3(iq)
  [iq] -> Iq/3(iq)
  [we] -> Id/4(we)
  [we] -> Iq/4(we)
  [awd] -> Id/5(du_d_z)
  [awq] -> Iq/5(du_q_z)

== system PMLSM_ThreeLoop_Simple/Control_Task_10kHz/Position_Loop ==
  x_ref_mm : Inport
  x_mm : Inport  Port=2
  pos_pi_reset : Inport  Port=3
  v_ff_pos : Inport  Port=4
  Trigger : TriggerPort  VariantControl=(inherit)
  Dead Zone : DeadZone  LowerValue=-Pos_deadband  UpperValue=+Pos_deadband
  Gain : Gain  Gain=Kp_pos
  Saturation : Saturate  UpperLimit=V_pos_max_mmps  LowerLimit=-V_pos_max_mmps
  Sum : Sum  Inputs=|+-
  Sum1 : Sum  Inputs=|++
  Terminator : Terminator
  v_ref_pos : Outport
  wires:
  x_ref_mm/1 -> Sum/1
  x_mm/1 -> Sum/2
  Sum/1 -> Dead Zone/1  "e_pos"
  Dead Zone/1 -> Gain/1
  Gain/1 -> Sum1/1
  v_ff_pos/1 -> Sum1/2
  Sum1/1 -> Saturation/1
  pos_pi_reset/1 -> Terminator/1
  Saturation/1 -> v_ref_pos/1  "obs_v_ref_pos"

== system PMLSM_ThreeLoop_Simple/Control_Task_10kHz/Reference_Manager ==
  iq_ref_normal : Inport
  v_ref_pos : Inport  Port=2
  Pos_Loop_EN : Inport  Port=3
  Close_Loop_EN : Inport  Port=4
  v_ref_cmd : Inport  Port=5
  id_ref_cmd : Inport  Port=6
  Iq_Test_Mode : Inport  Port=7
  iq_test_ref : Inport  Port=8
  Constant15 : Constant  Value=0
  Saturation : Saturate  UpperLimit=v_ref_max  LowerLimit=-v_ref_max
  Switch : Switch  Criteria=u2 > Threshold  Threshold=0.5  SaturateOnIntegerOverflow=off  InputSameDT=off
  Switch9 : Switch  Criteria=u2 > Threshold  Threshold=0.5  SaturateOnIntegerOverflow=off  InputSameDT=off
  v_ref_closed_sel : Switch  Criteria=u2 > Threshold  Threshold=0.5  SaturateOnIntegerOverflow=off  InputSameDT=off
  v_ref_set_slew_limiter : Subsystem
  id_ref : Outport
  iq_ref : Outport  Port=2
  v_ref : Outport  Port=3
  wires:
  Switch/1 -> iq_ref/1
  Switch9/1 -> v_ref/1
  Close_Loop_EN/1 -> Switch9/2
  iq_test_ref/1 -> Switch/1
  Iq_Test_Mode/1 -> Switch/2
  Constant15/1 -> Switch9/3
  iq_ref_normal/1 -> Switch/3
  id_ref_cmd/1 -> id_ref/1
  v_ref_set_slew_limiter/1(v_ref_set_limited) -> Saturation/1
  v_ref_pos/1 -> v_ref_closed_sel/1
  v_ref_closed_sel/1 -> v_ref_set_slew_limiter/1(v_ref_set)  "v_ref_closed"
  Pos_Loop_EN/1 -> v_ref_closed_sel/2
  Saturation/1 -> Switch9/1
  v_ref_cmd/1 -> v_ref_closed_sel/3

== system PMLSM_ThreeLoop_Simple/Control_Task_10kHz/Scheduler_10k_1k_100 ==
  note: position 计数链(/100)
  note: speed 计数链(/10)
  Add1 : Sum
  Add2 : Sum
  Constant1 : Constant
  Constant2 : Constant  Value=0
  Constant3 : Constant
  Constant4 : Constant  Value=0
  Logical Operator : Logic  AllPortsSameDT=off  OutDataTypeStr=boolean
  pos_cnt_hold_sel : Switch  Criteria=u2 > Threshold  Threshold=0.5  SaturateOnIntegerOverflow=off  InputSameDT=off
  pos_cnt_update_sel : Switch  Criteria=u2 > Threshold  Threshold=0.5  SaturateOnIntegerOverflow=off  InputSameDT=off
  pos_cnt_z : UnitDelay  SampleTime=-1
  pos_tc : simulink/Logic and Bit Operations/Compare To Constant  relop=>=  const=10  OutDataTypeStr=boolean
  spd_cnt_next_sel : Switch  Criteria=u2 > Threshold  Threshold=0.5  SaturateOnIntegerOverflow=off  InputSameDT=off
  spd_cnt_z : UnitDelay  SampleTime=-1
  spd_tc : simulink/Logic and Bit Operations/Compare To Constant  relop=>=  const=10  OutDataTypeStr=boolean
  speed_tick : Outport
  pos_tick : Outport  Port=2
  wires:
  spd_cnt_z/1 -> Add1/1
  spd_tc/1 -> speed_tick/1, Logical Operator/1, pos_cnt_hold_sel/2, spd_cnt_next_sel/2
  Constant1/1 -> Add1/2
  Constant2/1 -> spd_cnt_next_sel/1
  spd_cnt_next_sel/1 -> spd_cnt_z/1
  Add1/1 -> spd_cnt_next_sel/3, spd_tc/1  "spd_cnt_inc"
  pos_cnt_z/1 -> Add2/1, pos_cnt_hold_sel/3
  Constant3/1 -> Add2/2
  Add2/1 -> pos_cnt_update_sel/3, pos_tc/1  "pos_cnt_inc"
  pos_tc/1 -> Logical Operator/2, pos_cnt_update_sel/2
  Constant4/1 -> pos_cnt_update_sel/1
  pos_cnt_update_sel/1 -> pos_cnt_hold_sel/1  "pos_cnt_update_candidate"
  pos_cnt_hold_sel/1 -> pos_cnt_z/1
  Logical Operator/1 -> pos_tick/1

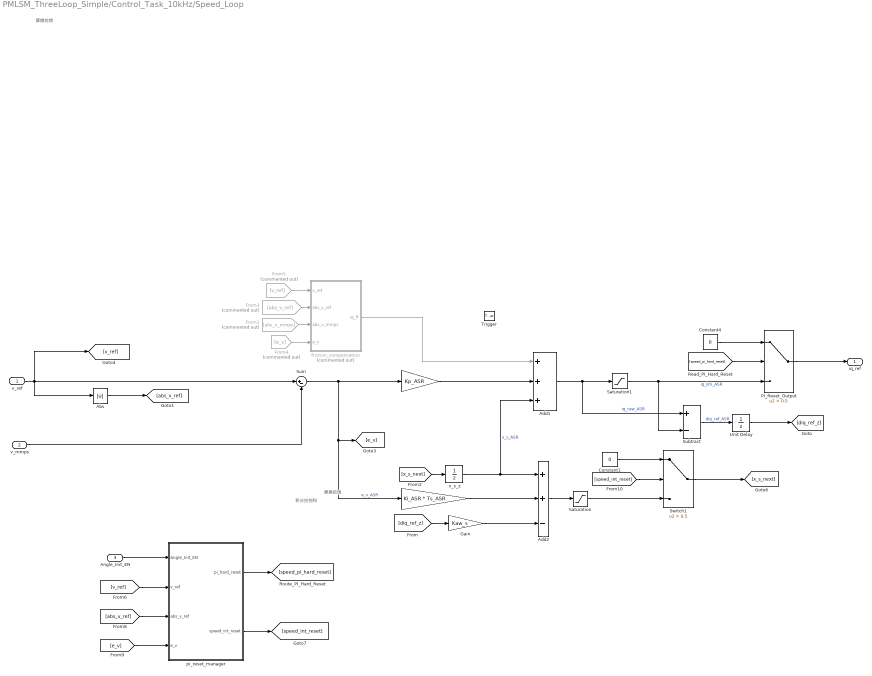
== system PMLSM_ThreeLoop_Simple/Control_Task_10kHz/Speed_Loop ==
  note: 摩擦前馈
  note: 积分抗饱和
  note: 摩擦前馈
  v_ref : Inport
  v_mmps : Inport  Port=2
  Angle_Init_EN : Inport  Port=3
  Trigger : TriggerPort  VariantControl=(inherit)
  " " : Gain  Gain=Ki_ASR * Ts_ASR
  "  " : Gain  Gain=Kp_ASR
  Abs : Abs  SaturateOnIntegerOverflow=off
  Add1 : Sum  Inputs=+++
  Add2 : Sum  Inputs=++-
  Constant1 : Constant  Value=0
  Constant4 : Constant  Value=0
  From1 : From  Commented=on  GotoTag=abs_v_mmps
  From3 : From  Commented=on  GotoTag=abs_v_ref
  From4 : From  Commented=on  GotoTag=e_v
  From5 : From  Commented=on  GotoTag=v_ref
  Gain : Gain  Gain=Kaw_s
  PI_Reset_Output : Switch  Criteria=u2 > Threshold  Threshold=0.5  SaturateOnIntegerOverflow=off  InputSameDT=off
  Saturation : Saturate  UpperLimit=Iq_int_limit  LowerLimit=-Iq_int_limit
  Saturation1 : Saturate  UpperLimit=Speed_loop_Iq_Limit  LowerLimit=-Speed_loop_Iq_Limit
  Subtract : Sum  Inputs=+-
  Sum : Sum  Inputs=|+-
  Switch1 : Switch  Criteria=u2 > Threshold  Threshold=0.5  SaturateOnIntegerOverflow=off  InputSameDT=off
  Unit Delay : UnitDelay  SampleTime=-1
  friction_compensation : Subsystem  Commented=on
  pi_reset_manager : Subsystem
  x_s_z : UnitDelay  SampleTime=-1
  iq_ref : Outport
  wires:
  Sum/1 -> [e_v], " "/1, "  "/1  "e_v_ASR"
  Add1/1 -> Subtract/1, Saturation1/1  "iq_raw_ASR"
  v_ref/1 -> Sum/1, Abs/1, [v_ref]
  Saturation1/1 -> PI_Reset_Output/3, Subtract/2  "iq_lim_ASR"
  [x_s_next] -> x_s_z/1
  Add2/1 -> Saturation/1
  Gain/1 -> Add2/3
  " "/1 -> Add2/2
  Subtract/1 -> Unit Delay/1  "diq_ref_ASR"
  Unit Delay/1 -> [diq_ref_z]
  [diq_ref_z] -> Gain/1
  Constant1/1 -> Switch1/1
  PI_Reset_Output/1 -> iq_ref/1
  Constant4/1 -> PI_Reset_Output/1
  "  "/1 -> Add1/2
  friction_compensation/1(iq_ff) -> Add1/1
  x_s_z/1 -> Add1/3, Add2/1  "x_s_ASR"
  From4/1 -> friction_compensation/4(e_v)
  From1/1 -> friction_compensation/3(abs_v_mmps)
  From3/1 -> friction_compensation/2(abs_v_ref)
  Abs/1 -> [abs_v_ref]
  Angle_Init_EN/1 -> pi_reset_manager/1(Angle_Init_EN)
  From5/1 -> friction_compensation/1(v_ref)
  [v_ref] -> pi_reset_manager/2(v_ref)
  [abs_v_ref] -> pi_reset_manager/3(abs_v_ref)
  [e_v] -> pi_reset_manager/4(e_v)
  [speed_pi_hard_reset] -> PI_Reset_Output/2
  pi_reset_manager/2(speed_int_reset) -> [speed_int_reset]
  pi_reset_manager/1(pi_hard_reset) -> [speed_pi_hard_reset]
  [speed_int_reset] -> Switch1/2
  Switch1/1 -> [x_s_next]
  Saturation/1 -> Switch1/3
  v_mmps/1 -> Sum/2

== system PMLSM_ThreeLoop_Simple/FPGA_HDL_Cosim/FPGA_Cosim_Monitor ==
  cmp_u_active : Inport
  cmp_v_active : Inport  Port=2
  cmp_w_active : Inport  Port=3
  accepted_sample_id : Inport  Port=4
  active_command_id : Inport  Port=5
  active_valid : Inport  Port=6
  needs_reset : Inport  Port=7
  fault_code : Inport  Port=8
  raw_duty_u : Inport  Port=9
  raw_duty_v : Inport  Port=10
  raw_duty_w : Inport  Port=11
  range_flags : Inport  Port=12
  FPGA_Interface_Log : ToWorkspace  VariableName=fpga_interface_monitor  SaveFormat=Timeseries  SampleTime=-1
  Pack : Mux  Inputs=12
  wires:
  cmp_u_active/1 -> Pack/1
  cmp_v_active/1 -> Pack/2
  cmp_w_active/1 -> Pack/3
  accepted_sample_id/1 -> Pack/4
  active_command_id/1 -> Pack/5
  active_valid/1 -> Pack/6
  needs_reset/1 -> Pack/7
  fault_code/1 -> Pack/8
  raw_duty_u/1 -> Pack/9
  raw_duty_v/1 -> Pack/10
  raw_duty_w/1 -> Pack/11
  range_flags/1 -> Pack/12
  Pack/1 -> FPGA_Interface_Log/1

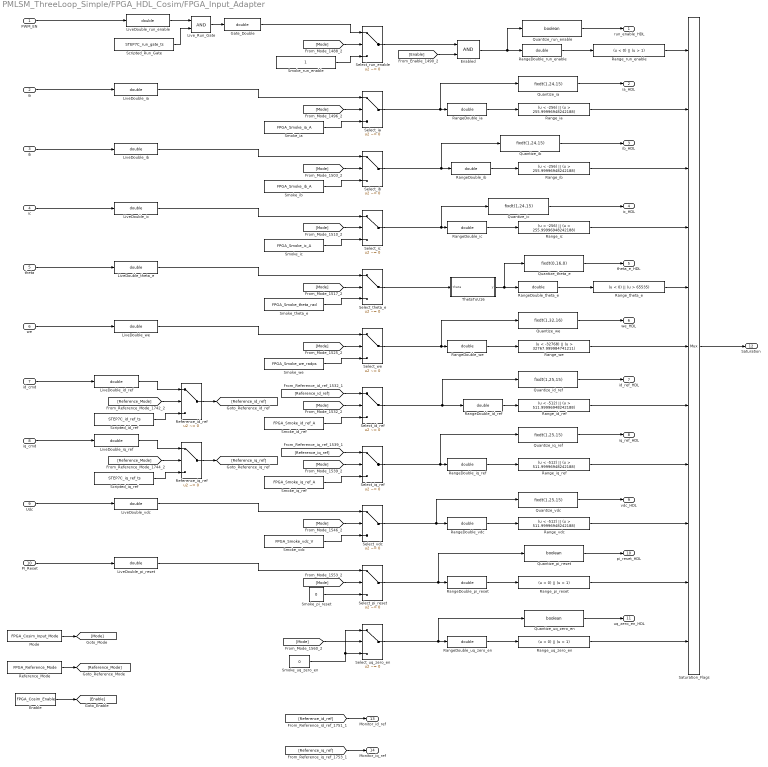
== system PMLSM_ThreeLoop_Simple/FPGA_HDL_Cosim/FPGA_Input_Adapter ==
  PWM_EN : Inport
  ia : Inport  Port=2
  ib : Inport  Port=3
  ic : Inport  Port=4
  theta : Inport  Port=5
  we : Inport  Port=6
  id_cmd : Inport  Port=7
  iq_cmd : Inport  Port=8
  Udc : Inport  Port=9
  PI_Reset : Inport  Port=10
  Enable : Constant  Value=FPGA_Cosim_Enable
  Enabled : Logic  AllPortsSameDT=off  OutDataTypeStr=boolean
  Gate_Double : DataTypeConversion  OutDataTypeStr=double  SaturateOnIntegerOverflow=off  RndMeth=Floor
  LiveDouble_ia : DataTypeConversion  OutDataTypeStr=double  SaturateOnIntegerOverflow=off  RndMeth=Floor
  LiveDouble_ib : DataTypeConversion  OutDataTypeStr=double  SaturateOnIntegerOverflow=off  RndMeth=Floor
  LiveDouble_ic : DataTypeConversion  OutDataTypeStr=double  SaturateOnIntegerOverflow=off  RndMeth=Floor
  LiveDouble_id_ref : DataTypeConversion  OutDataTypeStr=double  SaturateOnIntegerOverflow=off  RndMeth=Floor
  LiveDouble_iq_ref : DataTypeConversion  OutDataTypeStr=double  SaturateOnIntegerOverflow=off  RndMeth=Floor
  LiveDouble_pi_reset : DataTypeConversion  OutDataTypeStr=double  SaturateOnIntegerOverflow=off  RndMeth=Floor
  LiveDouble_run_enable : DataTypeConversion  OutDataTypeStr=double  SaturateOnIntegerOverflow=off  RndMeth=Floor
  LiveDouble_theta_e : DataTypeConversion  OutDataTypeStr=double  SaturateOnIntegerOverflow=off  RndMeth=Floor
  LiveDouble_vdc : DataTypeConversion  OutDataTypeStr=double  SaturateOnIntegerOverflow=off  RndMeth=Floor
  LiveDouble_we : DataTypeConversion  OutDataTypeStr=double  SaturateOnIntegerOverflow=off  RndMeth=Floor
  Live_Run_Gate : Logic  AllPortsSameDT=off  OutDataTypeStr=boolean
  Mode : Constant  Value=FPGA_Cosim_Input_Mode
  Quantize_ia : DataTypeConversion  OutDataTypeStr=fixdt(1,24,15)  RndMeth=Nearest
  Quantize_ib : DataTypeConversion  OutDataTypeStr=fixdt(1,24,15)  RndMeth=Nearest
  Quantize_ic : DataTypeConversion  OutDataTypeStr=fixdt(1,24,15)  RndMeth=Nearest
  Quantize_id_ref : DataTypeConversion  OutDataTypeStr=fixdt(1,25,15)  RndMeth=Nearest
  Quantize_iq_ref : DataTypeConversion  OutDataTypeStr=fixdt(1,25,15)  RndMeth=Nearest
  Quantize_pi_reset : DataTypeConversion  OutDataTypeStr=boolean  RndMeth=Nearest
  Quantize_run_enable : DataTypeConversion  OutDataTypeStr=boolean  RndMeth=Nearest
  Quantize_theta_e : DataTypeConversion  OutDataTypeStr=fixdt(0,16,0)  RndMeth=Nearest
  Quantize_uq_zero_en : DataTypeConversion  OutDataTypeStr=boolean  RndMeth=Nearest
  Quantize_vdc : DataTypeConversion  OutDataTypeStr=fixdt(1,25,15)  RndMeth=Nearest
  Quantize_we : DataTypeConversion  OutDataTypeStr=fixdt(1,32,16)  RndMeth=Nearest
  RangeDouble_ia : DataTypeConversion  OutDataTypeStr=double  SaturateOnIntegerOverflow=off  RndMeth=Floor
  RangeDouble_ib : DataTypeConversion  OutDataTypeStr=double  SaturateOnIntegerOverflow=off  RndMeth=Floor
  RangeDouble_ic : DataTypeConversion  OutDataTypeStr=double  SaturateOnIntegerOverflow=off  RndMeth=Floor
  RangeDouble_id_ref : DataTypeConversion  OutDataTypeStr=double  SaturateOnIntegerOverflow=off  RndMeth=Floor
  RangeDouble_iq_ref : DataTypeConversion  OutDataTypeStr=double  SaturateOnIntegerOverflow=off  RndMeth=Floor
  RangeDouble_pi_reset : DataTypeConversion  OutDataTypeStr=double  SaturateOnIntegerOverflow=off  RndMeth=Floor
  RangeDouble_run_enable : DataTypeConversion  OutDataTypeStr=double  SaturateOnIntegerOverflow=off  RndMeth=Floor
  RangeDouble_theta_e : DataTypeConversion  OutDataTypeStr=double  SaturateOnIntegerOverflow=off  RndMeth=Floor
  RangeDouble_uq_zero_en : DataTypeConversion  OutDataTypeStr=double  SaturateOnIntegerOverflow=off  RndMeth=Floor
  RangeDouble_vdc : DataTypeConversion  OutDataTypeStr=double  SaturateOnIntegerOverflow=off  RndMeth=Floor
  RangeDouble_we : DataTypeConversion  OutDataTypeStr=double  SaturateOnIntegerOverflow=off  RndMeth=Floor
  Range_ia : Fcn  Expr=(u < -256) || (u > 255.99996948242188)
  Range_ib : Fcn  Expr=(u < -256) || (u > 255.99996948242188)
  Range_ic : Fcn  Expr=(u < -256) || (u > 255.99996948242188)
  Range_id_ref : Fcn  Expr=(u < -512) || (u > 511.99996948242188)
  Range_iq_ref : Fcn  Expr=(u < -512) || (u > 511.99996948242188)
  Range_pi_reset : Fcn  Expr=(u < 0) || (u > 1)
  Range_run_enable : Fcn  Expr=(u < 0) || (u > 1)
  Range_theta_e : Fcn  Expr=(u < 0) || (u > 65535)
  Range_uq_zero_en : Fcn  Expr=(u < 0) || (u > 1)
  Range_vdc : Fcn  Expr=(u < -512) || (u > 511.99996948242188)
  Range_we : Fcn  Expr=(u < -32768) || (u > 32767.999984741211)
  Reference_Mode : Constant  Value=FPGA_Reference_Mode
  Reference_id_ref : Switch  Criteria=u2 ~= 0  SaturateOnIntegerOverflow=off  InputSameDT=off
  Reference_iq_ref : Switch  Criteria=u2 ~= 0  SaturateOnIntegerOverflow=off  InputSameDT=off
  Saturation_Flags : Mux  Inputs=11
  Scripted_Run_Gate : FromWorkspace  VariableName=STEP7C_run_gate_ts  SampleTime=FPGA_Cosim_Ts_s  Interpolate=off  OutputAfterFinalValue=Holding final value
  Scripted_id_ref : FromWorkspace  VariableName=STEP7C_id_ref_ts  SampleTime=FPGA_Cosim_Ts_s  Interpolate=off  OutputAfterFinalValue=Holding final value
  Scripted_iq_ref : FromWorkspace  VariableName=STEP7C_iq_ref_ts  SampleTime=FPGA_Cosim_Ts_s  Interpolate=off  OutputAfterFinalValue=Holding final value
  Select_ia : Switch  Criteria=u2 ~= 0  SaturateOnIntegerOverflow=off  InputSameDT=off
  Select_ib : Switch  Criteria=u2 ~= 0  SaturateOnIntegerOverflow=off  InputSameDT=off
  Select_ic : Switch  Criteria=u2 ~= 0  SaturateOnIntegerOverflow=off  InputSameDT=off
  Select_id_ref : Switch  Criteria=u2 ~= 0  SaturateOnIntegerOverflow=off  InputSameDT=off
  Select_iq_ref : Switch  Criteria=u2 ~= 0  SaturateOnIntegerOverflow=off  InputSameDT=off
  Select_pi_reset : Switch  Criteria=u2 ~= 0  SaturateOnIntegerOverflow=off  InputSameDT=off
  Select_run_enable : Switch  Criteria=u2 ~= 0  SaturateOnIntegerOverflow=off  InputSameDT=off
  Select_theta_e : Switch  Criteria=u2 ~= 0  SaturateOnIntegerOverflow=off  InputSameDT=off
  Select_uq_zero_en : Switch  Criteria=u2 ~= 0  SaturateOnIntegerOverflow=off  InputSameDT=off
  Select_vdc : Switch  Criteria=u2 ~= 0  SaturateOnIntegerOverflow=off  InputSameDT=off
  Select_we : Switch  Criteria=u2 ~= 0  SaturateOnIntegerOverflow=off  InputSameDT=off
  Smoke_ia : Constant  Value=FPGA_Smoke_ia_A  SampleTime=FPGA_Cosim_Ts_s
  Smoke_ib : Constant  Value=FPGA_Smoke_ib_A  SampleTime=FPGA_Cosim_Ts_s
  Smoke_ic : Constant  Value=FPGA_Smoke_ic_A  SampleTime=FPGA_Cosim_Ts_s
  Smoke_id_ref : Constant  Value=FPGA_Smoke_id_ref_A  SampleTime=FPGA_Cosim_Ts_s
  Smoke_iq_ref : Constant  Value=FPGA_Smoke_iq_ref_A  SampleTime=FPGA_Cosim_Ts_s
  Smoke_pi_reset : Constant  Value=0  SampleTime=FPGA_Cosim_Ts_s
  Smoke_run_enable : Constant  SampleTime=FPGA_Cosim_Ts_s
  Smoke_theta_e : Constant  Value=FPGA_Smoke_theta_rad  SampleTime=FPGA_Cosim_Ts_s
  Smoke_uq_zero_en : Constant  Value=0  SampleTime=FPGA_Cosim_Ts_s
  Smoke_vdc : Constant  Value=FPGA_Smoke_vdc_V  SampleTime=FPGA_Cosim_Ts_s
  Smoke_we : Constant  Value=FPGA_Smoke_we_radps  SampleTime=FPGA_Cosim_Ts_s
  ThetaToU16 : MATLAB Function  TreatAsAtomicUnit=on
  run_enable_HDL : Outport
  ia_HDL : Outport  Port=2
  ib_HDL : Outport  Port=3
  ic_HDL : Outport  Port=4
  theta_e_HDL : Outport  Port=5
  we_HDL : Outport  Port=6
  id_ref_HDL : Outport  Port=7
  iq_ref_HDL : Outport  Port=8
  vdc_HDL : Outport  Port=9
  pi_reset_HDL : Outport  Port=10
  uq_zero_en_HDL : Outport  Port=11
  Saturation : Outport  Port=12
  Monitor_id_ref : Outport  Port=13
  Monitor_iq_ref : Outport  Port=14
  wires:
  Quantize_run_enable/1 -> run_enable_HDL/1
  RangeDouble_run_enable/1 -> Range_run_enable/1
  LiveDouble_ib/1 -> Select_ib/1
  Smoke_ib/1 -> Select_ib/3
  Select_ib/1 -> Quantize_ib/1, RangeDouble_ib/1
  Quantize_ib/1 -> ib_HDL/1
  RangeDouble_ib/1 -> Range_ib/1
  Select_theta_e/1 -> ThetaToU16/1(theta)
  ThetaToU16/1(y) -> Quantize_theta_e/1, RangeDouble_theta_e/1
  Quantize_theta_e/1 -> theta_e_HDL/1
  RangeDouble_theta_e/1 -> Range_theta_e/1
  we/1 -> LiveDouble_we/1
  LiveDouble_we/1 -> Select_we/1
  Smoke_we/1 -> Select_we/3
  Select_we/1 -> Quantize_we/1, RangeDouble_we/1
  Quantize_we/1 -> we_HDL/1
  RangeDouble_we/1 -> Range_we/1
  iq_cmd/1 -> LiveDouble_iq_ref/1
  Select_iq_ref/1 -> RangeDouble_iq_ref/1, Quantize_iq_ref/1
  Quantize_iq_ref/1 -> iq_ref_HDL/1
  RangeDouble_iq_ref/1 -> Range_iq_ref/1
  Smoke_vdc/1 -> Select_vdc/3
  Select_vdc/1 -> Quantize_vdc/1, RangeDouble_vdc/1
  Quantize_vdc/1 -> vdc_HDL/1
  RangeDouble_vdc/1 -> Range_vdc/1
  PI_Reset/1 -> LiveDouble_pi_reset/1
  LiveDouble_pi_reset/1 -> Select_pi_reset/1
  Smoke_pi_reset/1 -> Select_pi_reset/3
  Select_pi_reset/1 -> RangeDouble_pi_reset/1, Quantize_pi_reset/1
  Quantize_pi_reset/1 -> pi_reset_HDL/1
  RangeDouble_pi_reset/1 -> Range_pi_reset/1
  Select_uq_zero_en/1 -> RangeDouble_uq_zero_en/1, Quantize_uq_zero_en/1
  Quantize_uq_zero_en/1 -> uq_zero_en_HDL/1
  RangeDouble_uq_zero_en/1 -> Range_uq_zero_en/1
  LiveDouble_iq_ref/1 -> Reference_iq_ref/1
  Scripted_iq_ref/1 -> Reference_iq_ref/3
  Scripted_Run_Gate/1 -> Live_Run_Gate/2
  Live_Run_Gate/1 -> Gate_Double/1
  [Enable] -> Enabled/2
  [Reference_Mode] -> Reference_iq_ref/2
  [Reference_Mode] -> Reference_id_ref/2
  [Mode] -> Select_uq_zero_en/2
  [Mode] -> Select_pi_reset/2
  [Mode] -> Select_vdc/2
  [Mode] -> Select_iq_ref/2
  [Mode] -> Select_id_ref/2
  [Mode] -> Select_we/2
  [Mode] -> Select_theta_e/2
  [Mode] -> Select_ic/2
  [Mode] -> Select_ib/2
  [Mode] -> Select_ia/2
  [Mode] -> Select_run_enable/2
  Gate_Double/1 -> Select_run_enable/1
  LiveDouble_run_enable/1 -> Live_Run_Gate/1
  Scripted_id_ref/1 -> Reference_id_ref/3
  Reference_Mode/1 -> [Reference_Mode]
  LiveDouble_id_ref/1 -> Reference_id_ref/1
  Saturation_Flags/1 -> Saturation/1
  Range_uq_zero_en/1 -> Saturation_Flags/11
  Smoke_uq_zero_en/1 -> Select_uq_zero_en/3, Select_uq_zero_en/1
  Range_pi_reset/1 -> Saturation_Flags/10
  Range_vdc/1 -> Saturation_Flags/9
  LiveDouble_vdc/1 -> Select_vdc/1
  Udc/1 -> LiveDouble_vdc/1
  Range_iq_ref/1 -> Saturation_Flags/8
  Smoke_iq_ref/1 -> Select_iq_ref/3
  Range_id_ref/1 -> Saturation_Flags/7
  RangeDouble_id_ref/1 -> Range_id_ref/1
  Quantize_id_ref/1 -> id_ref_HDL/1
  Select_id_ref/1 -> Quantize_id_ref/1, RangeDouble_id_ref/1
  Smoke_id_ref/1 -> Select_id_ref/3
  Range_we/1 -> Saturation_Flags/6
  Range_theta_e/1 -> Saturation_Flags/5
  Smoke_theta_e/1 -> Select_theta_e/3
  LiveDouble_theta_e/1 -> Select_theta_e/1
  theta/1 -> LiveDouble_theta_e/1
  Range_ic/1 -> Saturation_Flags/4
  RangeDouble_ic/1 -> Range_ic/1
  Quantize_ic/1 -> ic_HDL/1
  Select_ic/1 -> Quantize_ic/1, RangeDouble_ic/1
  Smoke_ic/1 -> Select_ic/3
  LiveDouble_ic/1 -> Select_ic/1
  ic/1 -> LiveDouble_ic/1
  Range_ib/1 -> Saturation_Flags/3
  ib/1 -> LiveDouble_ib/1
  Range_ia/1 -> Saturation_Flags/2
  RangeDouble_ia/1 -> Range_ia/1
  Quantize_ia/1 -> ia_HDL/1
  Select_ia/1 -> Quantize_ia/1, RangeDouble_ia/1
  Smoke_ia/1 -> Select_ia/3
  LiveDouble_ia/1 -> Select_ia/1
  ia/1 -> LiveDouble_ia/1
  Range_run_enable/1 -> Saturation_Flags/1
  Enabled/1 -> Quantize_run_enable/1, RangeDouble_run_enable/1
  Enable/1 -> [Enable]
  Select_run_enable/1 -> Enabled/1
  Smoke_run_enable/1 -> Select_run_enable/3
  Mode/1 -> [Mode]
  PWM_EN/1 -> LiveDouble_run_enable/1
  [Reference_iq_ref] -> Monitor_iq_ref/1
  [Reference_iq_ref] -> Select_iq_ref/1
  [Reference_id_ref] -> Select_id_ref/1
  [Reference_id_ref] -> Monitor_id_ref/1
  id_cmd/1 -> LiveDouble_id_ref/1
  Reference_id_ref/1 -> [Reference_id_ref]
  Reference_iq_ref/1 -> [Reference_iq_ref]

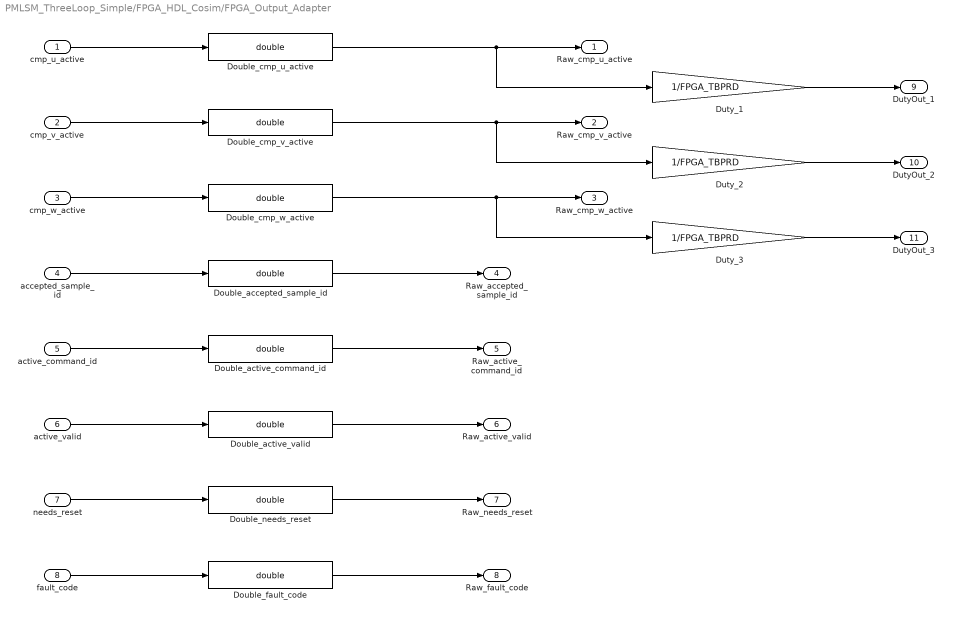
== system PMLSM_ThreeLoop_Simple/FPGA_HDL_Cosim/FPGA_Output_Adapter ==
  cmp_u_active : Inport
  cmp_v_active : Inport  Port=2
  cmp_w_active : Inport  Port=3
  accepted_sample_id : Inport  Port=4
  active_command_id : Inport  Port=5
  active_valid : Inport  Port=6
  needs_reset : Inport  Port=7
  fault_code : Inport  Port=8
  Double_accepted_sample_id : DataTypeConversion  OutDataTypeStr=double  SaturateOnIntegerOverflow=off  RndMeth=Floor
  Double_active_command_id : DataTypeConversion  OutDataTypeStr=double  SaturateOnIntegerOverflow=off  RndMeth=Floor
  Double_active_valid : DataTypeConversion  OutDataTypeStr=double  SaturateOnIntegerOverflow=off  RndMeth=Floor
  Double_cmp_u_active : DataTypeConversion  OutDataTypeStr=double  SaturateOnIntegerOverflow=off  RndMeth=Floor
  Double_cmp_v_active : DataTypeConversion  OutDataTypeStr=double  SaturateOnIntegerOverflow=off  RndMeth=Floor
  Double_cmp_w_active : DataTypeConversion  OutDataTypeStr=double  SaturateOnIntegerOverflow=off  RndMeth=Floor
  Double_fault_code : DataTypeConversion  OutDataTypeStr=double  SaturateOnIntegerOverflow=off  RndMeth=Floor
  Double_needs_reset : DataTypeConversion  OutDataTypeStr=double  SaturateOnIntegerOverflow=off  RndMeth=Floor
  Duty_1 : Gain  Gain=1/FPGA_TBPRD
  Duty_2 : Gain  Gain=1/FPGA_TBPRD
  Duty_3 : Gain  Gain=1/FPGA_TBPRD
  Raw_cmp_u_active : Outport
  Raw_cmp_v_active : Outport  Port=2
  Raw_cmp_w_active : Outport  Port=3
  Raw_accepted_sample_id : Outport  Port=4
  Raw_active_command_id : Outport  Port=5
  Raw_active_valid : Outport  Port=6
  Raw_needs_reset : Outport  Port=7
  Raw_fault_code : Outport  Port=8
  DutyOut_1 : Outport  Port=9
  DutyOut_2 : Outport  Port=10
  DutyOut_3 : Outport  Port=11
  wires:
  cmp_u_active/1 -> Double_cmp_u_active/1
  Double_cmp_u_active/1 -> Duty_1/1, Raw_cmp_u_active/1
  Duty_1/1 -> DutyOut_1/1
  cmp_v_active/1 -> Double_cmp_v_active/1
  Double_cmp_v_active/1 -> Duty_2/1, Raw_cmp_v_active/1
  Duty_2/1 -> DutyOut_2/1
  cmp_w_active/1 -> Double_cmp_w_active/1
  Double_cmp_w_active/1 -> Raw_cmp_w_active/1, Duty_3/1
  Duty_3/1 -> DutyOut_3/1
  accepted_sample_id/1 -> Double_accepted_sample_id/1
  Double_accepted_sample_id/1 -> Raw_accepted_sample_id/1
  active_command_id/1 -> Double_active_command_id/1
  Double_active_command_id/1 -> Raw_active_command_id/1
  active_valid/1 -> Double_active_valid/1
  Double_active_valid/1 -> Raw_active_valid/1
  needs_reset/1 -> Double_needs_reset/1
  Double_needs_reset/1 -> Raw_needs_reset/1
  fault_code/1 -> Double_fault_code/1
  Double_fault_code/1 -> Raw_fault_code/1

== system PMLSM_ThreeLoop_Simple/FPGA_HDL_Cosim/HDL_Backend_Variant ==
  In1 : Inport
  In2 : Inport  Port=2
  In3 : Inport  Port=3
  In4 : Inport  Port=4
  In5 : Inport  Port=5
  In6 : Inport  Port=6
  In7 : Inport  Port=7
  In8 : Inport  Port=8
  In9 : Inport  Port=9
  In10 : Inport  Port=10
  In11 : Inport  Port=11
  FPGA_Disabled : Subsystem  VariantControl=V_Backend_Legacy
  FPGA_Enabled : Subsystem  VariantControl=V_Backend_FPGA
  Out1 : Outport
  Out2 : Outport  Port=2
  Out3 : Outport  Port=3
  Out4 : Outport  Port=4
  Out5 : Outport  Port=5
  Out6 : Outport  Port=6
  Out7 : Outport  Port=7
  Out8 : Outport  Port=8
